simulink model "gNautilus_model_LSL_32_Thomas_22a"  (R2022b)
settings: Solver=ode45  StartTime=0.0  StopTime=inf  RelTol=1e-3
model workspace (MAT data in the model file):
  cfg_native : object (value not decoded)
  en_add_channels = 69
  host_ip = 2130706433
  host_port = 50223
  local_ip = 2130706433
  local_port = 50224
  num_en_channels = 14
  num_samples = 8
  sample_rate = 250
  serial_number = 'NB-2015.02.05'
undefined symbols (not defined in the file or in its folder): NB
libraries: instrumentlib x1, gNautilusLib x1, gNautilusTools x1
settings Model: Creator=gtec  LastModifiedBy=tohim
settings SolverCC: AlgebraicLoopSolver=TrustRegion
settings DataIOCC: ReturnWorkspaceOutputs=off
settings OptimizationCC: LifeSpan=inf
settings DebuggingCC: UnconnectedInputMsg=warning  UnconnectedOutputMsg=warning  UnconnectedLineMsg=warning  SFExecutionAtInitializationDiag=none  SFMachineParentedDataDiag=warning  ArithmeticOperatorsInVariantConditions=warning
settings HardwareCC: ProdBitPerSizeT=32  ProdBitPerPtrDiffT=32  ProdWordSize=32  ProdHWDeviceType=Specified
settings ModelReferenceCC: EnableRefExpFcnMdlSchedulingChecks=on
settings SFSimCC: SimUseLocalCustomCode=off  CustomCodeUndefinedFunction=UseInterfaceOnly
settings RTWCC: RTWUseLocalCustomCode=off
settings CodeAppCC: StateflowObjectComments=on

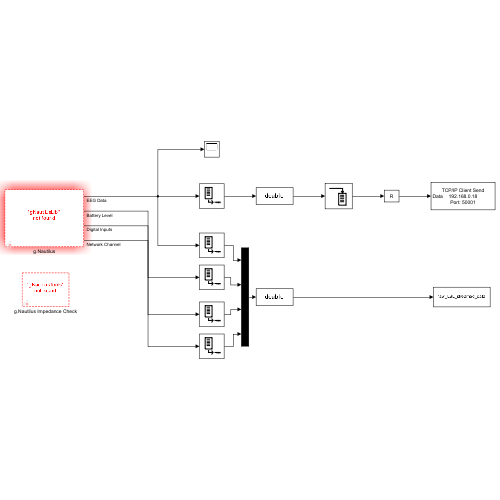
[thumbnail: Simulink's stored preview of the top-level diagram]
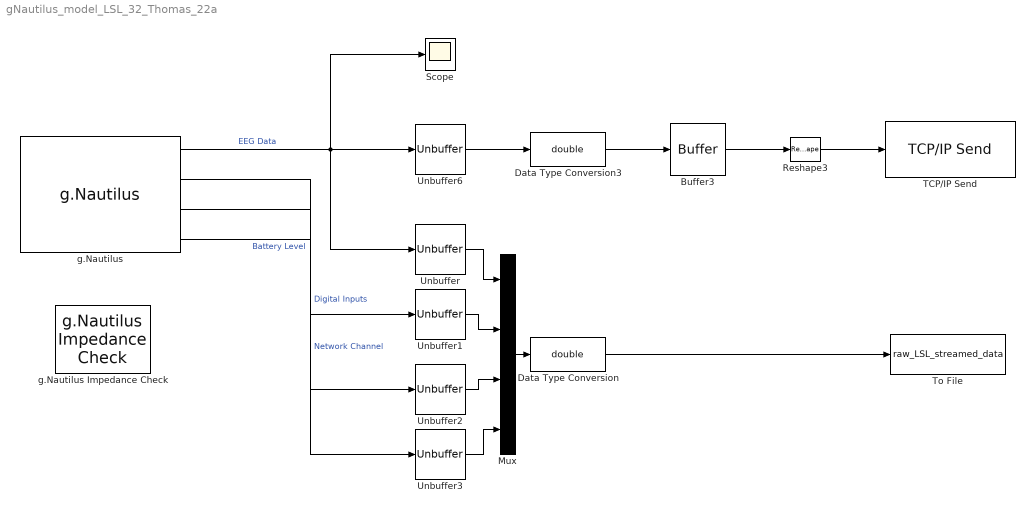
== system gNautilus_model_LSL_32_Thomas_22a ==
  Buffer3 : Buffer  N=1000  V=500  OutputFrames=off
  Data Type Conversion : DataTypeConversion  OutDataTypeStr=double  SaturateOnIntegerOverflow=off  RndMeth=Floor
  Data Type Conversion3 : DataTypeConversion  OutDataTypeStr=double  SaturateOnIntegerOverflow=off  RndMeth=Floor
  Mux : Mux
  Reshape3 : Reshape  OutputDimensionality=Customize  OutputDimensions=[14000,1]
  Scope : Scope
  TCP/IP Send : instrumentlib/TCP//IP Send  Host=192.168.0.18  Port=50001  ByteOrder=little-endian  EnableBlockingMode=on  Timeout=120  TransferDelay=off  SimulateUsing=Interpreted execution
  To File : ToFile  Filename=raw_LSL_streamed_data  MatrixName=y_n
  Unbuffer{,1..3,6} (5 alike) : Unbuffer
  g.Nautilus : gNautilusLib/g.Nautilus  Tag=g.Nautilus  Description=Operates a g.Nautilus device and provides acquired data on its outputs.  sample_rate=250  local_ip=2130706433  local_port=50224  host_ip=2130706433  host_port=50223  serial_number=NB-2015.02.05  num_samples=8  num_en_channels=14  add_channels=69
  g.Nautilus Impedance Check : gNautilusTools/g.Nautilus Impedance Check
  wires:
  g.Nautilus/1 -> Unbuffer/1, Unbuffer6/1, Scope/1  "EEG Data"
  Data Type Conversion/1 -> To File/1
  g.Nautilus/4 -> Unbuffer3/1  "Network Channel"
  g.Nautilus/2 -> Unbuffer1/1  "Battery Level"
  Unbuffer/1 -> Mux/1
  g.Nautilus/3 -> Unbuffer2/1  "Digital Inputs"
  Mux/1 -> Data Type Conversion/1
  Unbuffer1/1 -> Mux/2
  Unbuffer2/1 -> Mux/3
  Unbuffer3/1 -> Mux/4
  Unbuffer6/1 -> Data Type Conversion3/1
  Buffer3/1 -> Reshape3/1
  Reshape3/1 -> TCP/IP Send/1
  Data Type Conversion3/1 -> Buffer3/1
